simulink model "lvjy"  (R2019b)
settings: Solver=FixedStepAuto  StartTime=0.0  StopTime=10.0  FixedStep=0.004  RelTol=1e-3
values from neighbouring files (symbols this model uses):
  wn = 2*pi*F_Hz    (= 219.911485751)    [filter_2.m]
  zuni = 0.707    [filter_2.m]
settings Model: Creator=a4327  LastModifiedBy=a4327

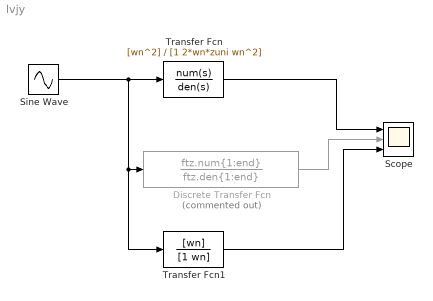
== system lvjy ==
  Discrete Transfer Fcn : DiscreteTransferFcn  Commented=on  Numerator=ftz.num{1:end}  Denominator=ftz.den{1:end}
  Scope : Scope  NumInputPorts=3
  Sine Wave : Sin  Frequency=20  SampleTime=0
  Transfer Fcn : TransferFcn  Numerator=[wn^2]  Denominator=[1 2*wn*zuni wn^2]
  Transfer Fcn1 : TransferFcn  Numerator=[wn]  Denominator=[1 wn]
  wires:
  Sine Wave/1 -> Transfer Fcn1/1, Discrete Transfer Fcn/1, Transfer Fcn/1
  Discrete Transfer Fcn/1 -> Scope/2
  Transfer Fcn/1 -> Scope/1
  Transfer Fcn1/1 -> Scope/3
